simulink subsystem "lqr_3dof"  (R2025b)
settings: Solver=VariableStepAuto  StartTime=0.0  StopTime=10.0  RelTol=1e-3
values from neighbouring files (symbols this model uses):
  K_free_rot = K_free_rot_erw(1:3, 1:6)    [params.m]
  Ki_free_rot = K_free_rot_erw(1:3, 7:9)    [params.m]
  S_free_rot = -inv(C_rot*inv((A_free_rot-B_rot*K_free_rot))* B_rot)    [params.m]
settings Model: Creator=schwmaxi  LastModifiedBy=schwmaxi

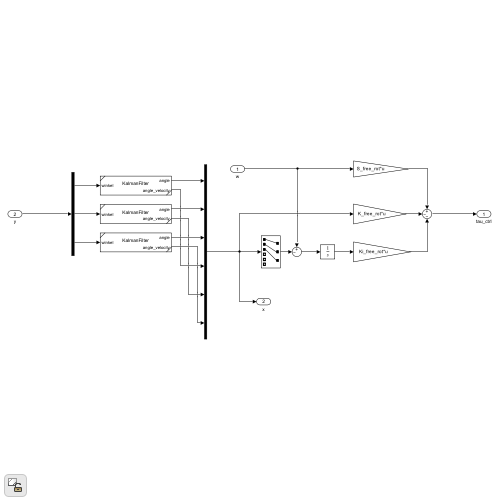
[thumbnail: Simulink's stored preview of the top-level diagram]
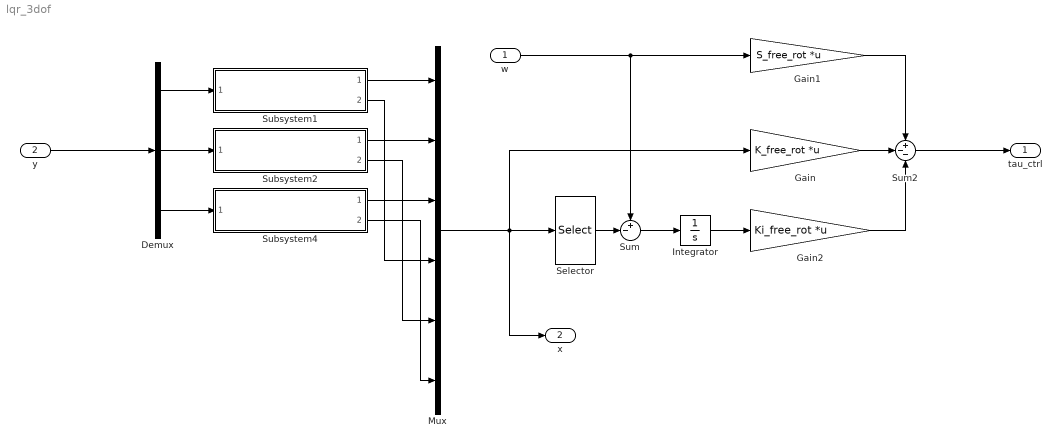
== system lqr_3dof ==
  w : Inport  OutDataTypeStr=double  PortDimensions=3  SampleTime=0
  y : Inport  Port=2  OutDataTypeStr=double  PortDimensions=3  SampleTime=0
  Demux : Demux  Outputs=3
  Gain : Gain  Gain=K_free_rot  Multiplication=Matrix(K*u)
  Gain1 : Gain  Gain=S_free_rot  Multiplication=Matrix(K*u)
  Gain2 : Gain  Gain=Ki_free_rot  Multiplication=Matrix(K*u)
  Integrator : Integrator
  Mux : Mux  Inputs=6
  Selector : Selector  InputPortWidth=6  IndexOptions=Index vector (dialog)  Indices=[1 2 3]  OutputSizes=1
  Subsystem1 : Subsystem  ReferencedSubsystem=KalmanFilter
  Subsystem2 : Subsystem  ReferencedSubsystem=KalmanFilter
  Subsystem4 : Subsystem  ReferencedSubsystem=KalmanFilter
  Sum : Sum  Inputs=+-|
  Sum2 : Sum  Inputs=+--
  tau_ctrl : Outport
  x : Outport  Port=2
  wires:
  Gain/1 -> Sum2/2
  Gain2/1 -> Sum2/3
  Integrator/1 -> Gain2/1
  Selector/1 -> Sum/2
  Sum/1 -> Integrator/1
  Demux/3 -> Subsystem4/1
  Demux/2 -> Subsystem2/1
  Demux/1 -> Subsystem1/1
  y/1 -> Demux/1
  Subsystem1/1 -> Mux/1
  Mux/1 -> Gain/1, Selector/1, x/1
  Subsystem1/2 -> Mux/4
  Subsystem4/2 -> Mux/6
  Subsystem2/1 -> Mux/2
  Subsystem4/1 -> Mux/3
  Subsystem2/2 -> Mux/5
  Sum2/1 -> tau_ctrl/1
  Gain1/1 -> Sum2/1
  w/1 -> Sum/1, Gain1/1
